simulink model "frft_qpsk_transceiver"  (R2025a)
settings: Solver=FixedStepDiscrete  StartTime=0.0  StopTime=1  RelTol=1e-3
PreLoadFcn:
  | % Add paths
  | addpath("dvb-s2/")
  | addpath("frft_filtering/")
  | addpath("gse")
  | 
  | 
  | 
  | 
  | setTxBurstLength = 10000;
  | txtmsg = ['Zynq radio HW/SW Co-design ÞÞÞÞ']; % Use only printable characters
  | 
  | %------------------------------------------------------------------------------------------------------
  | if ~isequal(size(txtmsg),[1 31])
  |     error('txtmsg must contain 31 characters');
  | end
  | 
  | [dataBits,msg] = zynqRadioHWSWQPSKgenHelloworldMsg(20); % generate 20 msgs for LUT
  | msgLUT = uint8(msg);
  | dataBitsLUT = dataBits(:);
  | Rsym                = 25e3;%1.92e6;
  | Config = zynqRadioHWSWQPSKTxRxParameters;
  | fs = Rsym*Config.SamplesPerSymbol;
  | word = [txtmsg newline];  % append a new line character to txtmsg
  | 
  | % The highest clock rate is 16 times the message character rate.
  | % As the message characters are fed at highest clock to FPGA
  | % repeat each character 16 times to maintain the message rate.
  | word = repelem(word.',16,1);
  | repeatTimes = ceil(setTxBurstLength/length(word));
  | inpData = complex(repmat(uint8(word),repeatTimes,1));
  | inUseTxBurstLength = length(inpData);
PostLoadFcn:
  | hScopeConfig = get_param([gcs '/HDL_QPSK/QPSK Tx Channel QPSK Rx/QPSK Rx/Frequency and Time Synchronizer/Symbol Synchronizer/No HDL/QPSK Receiver Eye Diagram'],'ScopeConfiguration');
  | hScopeConfig.OpenAtSimulationStart = false;
  | hScopeConfig.Visible = false;
  | clear hScopeConfig
InitFcn:
  | setTxBurstLength = 10000;
  | txtmsg = ['Zynq radio HW/SW Co-design ÞÞÞÞ']; % Use only printable characters
  | 
  | %------------------------------------------------------------------------------------------------------
  | if ~isequal(size(txtmsg),[1 31])
  |     error('txtmsg must contain 31 characters');
  | end
  | 
  | [dataBits,msg] = zynqRadioHWSWQPSKgenHelloworldMsg(20); % generate 20 msgs for LUT
  | msgLUT = uint8(msg);
  | dataBitsLUT = dataBits(:);
  | Rsym                = 25e3;%1.92e6;
  | Config = zynqRadioHWSWQPSKTxRxParameters;
  | fs = Rsym*Config.SamplesPerSymbol;
  | word = [txtmsg newline];  % append a new line character to txtmsg
  | 
  | % The highest clock rate is 16 times the message character rate.
  | % As the message characters are fed at highest clock to FPGA
  | % repeat each character 16 times to maintain the message rate.
  | word = repelem(word.',16,1);
  | repeatTimes = ceil(setTxBurstLength/length(word));
  | inpData = complex(repmat(uint8(word),repeatTimes,1));
  | inUseTxBurstLength = length(inpData);
undefined symbols (not defined in the file or in its folder): Add, dspblkCoreblockFVToolHelper, gcbh, Shift, unicode2native
libraries: hdlsllib x120, simulink x39, commseqgen3 x8, dsphdlsigops2 x4, whdledac x4, dsphdlfiltering2 x3, whdlutilities x3, dsphdlxfrm2 x2, dsphdlmathfun2 x2, commdigbbndpm3 x2, commchan3 x1, whdlmod x1
(part 5 of 5)

== system frft_qpsk_transceiver/Model Parameters/HDL_QPSK/QPSK Tx Channel QPSK Rx/QPSK Rx/Frequency and Time Synchronizer/Symbol Synchronizer/Rate Handle/FIFO ==
  in : Inport
  push : Inport  Port=2
  pop : Inport  Port=3
  reset : Inport  Port=4
  Delay1 : Delay  DelayLength=1
  Pop Counter : hdlsllib/Sources/HDL Counter  CountType=Count limited  CountInit=0  CountStep=1  CountMax=fifoSize -1  CountFromType=Initial value  CountFrom=0  CountResetPort=on  CountLoadPort=off  CountEnbPort=on  CountDirPort=off  CountHitOutputPort=off  CountDataType=Unsigned  CountWordLen=nextpow2(fifoSize)  CountFracLen=0  CountSampTime=1
  Push Counter : hdlsllib/Sources/HDL Counter  CountType=Count limited  CountInit=0  CountStep=1  CountMax=fifoSize -1  CountFromType=Initial value  CountFrom=0  CountResetPort=on  CountLoadPort=off  CountEnbPort=on  CountDirPort=off  CountHitOutputPort=off  CountDataType=Unsigned  CountWordLen=nextpow2(fifoSize)  CountFracLen=0  CountSampTime=1
  Simple Dual Port RAM : hdlsllib/HDL RAMs/Simple Dual Port RAM  ram_size=nextpow2(fifoSize)
  Validate Input Push Pop : Subsystem
  out : Outport
  numEntries : Outport  Port=2
  validPop : Outport  Port=3
  wires:
  Delay1/1 -> Push Counter/1, Pop Counter/1
  in/1 -> Simple Dual Port RAM/1
  reset/1 -> Validate Input Push Pop/1(rst), Delay1/1
  Validate Input Push Pop/2(valid pop) -> Pop Counter/2, validPop/1
  Validate Input Push Pop/1(valid push) -> Push Counter/2, Simple Dual Port RAM/3
  pop/1 -> Validate Input Push Pop/3(pop)
  push/1 -> Validate Input Push Pop/2(push)
  Pop Counter/1 -> Simple Dual Port RAM/4
  Push Counter/1 -> Simple Dual Port RAM/2
  Simple Dual Port RAM/1 -> out/1
  Validate Input Push Pop/3(numEntries) -> numEntries/1

== system frft_qpsk_transceiver/Model Parameters/HDL_QPSK/QPSK Tx Channel QPSK Rx/QPSK Tx/Bit Packetizer/Data Bits FIFO/No HDL/No HDL ==
  push : Inport
  full : Inport  Port=2
  ncount : Inport  Port=3
  empty : Inport  Port=4
  pop : Inport  Port=5
  Assertion : Assertion
  Assertion1 : Assertion
  Display : Display
  Logical Operator : Logic  Operator=NAND  AllPortsSameDT=off  OutDataTypeStr=boolean
  Logical Operator1 : Logic  Operator=NAND  AllPortsSameDT=off  OutDataTypeStr=boolean
  wires:
  Logical Operator1/1 -> Assertion1/1
  ncount/1 -> Display/1
  Logical Operator/1 -> Assertion/1
  pop/1 -> Logical Operator1/2
  full/1 -> Logical Operator/2
  empty/1 -> Logical Operator1/1
  push/1 -> Logical Operator/1

== system frft_qpsk_transceiver/Model Parameters/HDL_QPSK/QPSK Tx Channel QPSK Rx/QPSK Rx/Frequency and Time Synchronizer/Coarse Frequency Compensator/Coarse Frequency Estimator/Integrator/Reset Generator ==
  validIn : Inport
  Compare To Constant : simulink/Logic and Bit Operations/Compare To Constant  relop===  const=integAvgLen  OutDataTypeStr=boolean
  Delay1 : Delay  DelayLength=1
  Delay5 : Delay  DelayLength=1
  HDL Counter : hdlsllib/Sources/HDL Counter  CountType=Count limited  CountInit=0  CountStep=1  CountMax=integAvgLen  CountFromType=Initial value  CountFrom=0  CountResetPort=off  CountLoadPort=off  CountEnbPort=on  CountDirPort=off  CountHitOutputPort=off  CountDataType=Unsigned  CountWordLen=nextpow2(integAvgLen + 1)  CountFracLen=0  CountSampTime=1
  Logical Operator : Logic  AllPortsSameDT=off  OutDataTypeStr=boolean
  reset : Outport
  wires:
  Delay1/1 -> Logical Operator/1
  Delay5/1 -> Compare To Constant/1
  Logical Operator/1 -> reset/1
  validIn/1 -> HDL Counter/1, Delay1/1
  Compare To Constant/1 -> Logical Operator/2
  HDL Counter/1 -> Delay5/1

== system frft_qpsk_transceiver/Model Parameters/HDL_QPSK/QPSK Tx Channel QPSK Rx/QPSK Rx/Frequency and Time Synchronizer/PL Data Descrambler/PL Data Descrambler/PL Scrambler Gold Sequence Generator/Subsystem ==
  note: The initial output of these outports are set to 0 as this is an enabled subsystem
  reset : Inport
  Enable : EnablePort
  X PN Generator M_n : commseqgen3/PN Sequence Generator  poly='z^18+z^7+1'  ini_sta=[zeros(1,17) 1]  outBitMaskSource=Dialog parameter  shift=n  outVarSiz=off  maxOutSizeMode=Dialog parameter  maxOutSize=[10 1]  Ts=-1  sampPerFrame=1  reset=on  bitPackedOutputs=off  outDataType=boolean  numPackedBits=8  bitPackDataSigned=off  bitPackedOutDType=double
  X PN Generator M_nplus131072 : commseqgen3/PN Sequence Generator  poly='z^18+z^7+1'  ini_sta=[zeros(1,17) 1]  outBitMaskSource=Dialog parameter  shift=n+131072  outVarSiz=off  maxOutSizeMode=Dialog parameter  maxOutSize=[10 1]  Ts=-1  sampPerFrame=1  reset=on  bitPackedOutputs=off  outDataType=boolean  numPackedBits=8  bitPackDataSigned=off  bitPackedOutDType=double
  Y PN Generator M_0 : commseqgen3/PN Sequence Generator  poly='z^18 + z^10 + z^7 + z^5 + 1'  ini_sta=ones(1,18)  outBitMaskSource=Dialog parameter  shift=0  outVarSiz=off  maxOutSizeMode=Dialog parameter  maxOutSize=[10 1]  Ts=-1  sampPerFrame=1  reset=on  bitPackedOutputs=off  outDataType=boolean  numPackedBits=8  bitPackDataSigned=off  bitPackedOutDType=double
  Y PN Generator M_131072 : commseqgen3/PN Sequence Generator  poly='z^18 + z^10 + z^7 + z^5 + 1'  ini_sta=ones(1,18)  outBitMaskSource=Dialog parameter  shift=131072  outVarSiz=off  maxOutSizeMode=Dialog parameter  maxOutSize=[10 1]  Ts=-1  sampPerFrame=1  reset=on  bitPackedOutputs=off  outDataType=boolean  numPackedBits=8  bitPackDataSigned=off  bitPackedOutDType=double
  xMnp131072 : Outport  InitialOutput=0
  yM131072 : Outport  Port=2  InitialOutput=0
  xMn : Outport  Port=3  InitialOutput=0
  yM0 : Outport  Port=4  InitialOutput=0
  wires:
  X PN Generator M_nplus131072/1 -> xMnp131072/1
  Y PN Generator M_0/1 -> yM0/1
  reset/1 -> X PN Generator M_nplus131072/1, Y PN Generator M_0/1, X PN Generator M_n/1, Y PN Generator M_131072/1
  X PN Generator M_n/1 -> xMn/1
  Y PN Generator M_131072/1 -> yM131072/1

== system frft_qpsk_transceiver/Model Parameters/HDL_QPSK/QPSK Tx Channel QPSK Rx/QPSK Rx/Frequency and Time Synchronizer/Phase Ambiguity Estimation and Correction/Phase Ambiguity Corrector/Reciprocal/Function Impl ==
  switch : Inport
  LUTAddr : Inport  Port=2
  Delay{6..8,10,15..16} (6 alike) : Delay
  Delay9 : Delay  DelayLength=1
  LUT1 : LookupNDDirect  NumberOfTableDimensions=1  Table=LUT(:,1)  DiagnosticForOutOfRangeInput=Error
  LUT2 : LookupNDDirect  NumberOfTableDimensions=1  Table=LUT(:,2)  DiagnosticForOutOfRangeInput=Error
  Multiport Switch : MultiPortSwitch  DataPortOrder=Zero-based contiguous  Inputs=2  zeroidx=on  SaturateOnIntegerOverflow=off  InputSameDT=off
  functionValues : Outport
  wires:
  Multiport Switch/1 -> Delay9/1
  Delay6/1 -> LUT1/1
  Delay7/1 -> LUT2/1
  Delay8/1 -> Delay10/1
  switch/1 -> Delay8/1
  LUT1/1 -> Delay16/1
  LUT2/1 -> Delay15/1
  Delay9/1 -> functionValues/1
  Delay10/1 -> Multiport Switch/1
  Delay16/1 -> Multiport Switch/3
  Delay15/1 -> Multiport Switch/2
  LUTAddr/1 -> Delay6/1, Delay7/1

== system frft_qpsk_transceiver/Model Parameters/HDL_QPSK/QPSK Tx Channel QPSK Rx/QPSK Rx/Frequency and Time Synchronizer/Preamble Detector/Timing Adjust/No HDL/No HDL ==
  timingOffset : Inport
  Enable : EnablePort
  Data Type Conversion : DataTypeConversion  OutDataTypeStr=double  SaturateOnIntegerOverflow=off  RndMeth=Floor
  To Workspace : ToWorkspace  VariableName=simTimingOffset  SampleTime=-1
      settings: Save2DSignal=2-D array (concatenate along first dimension)
  wires:
  Data Type Conversion/1 -> To Workspace/1
  timingOffset/1 -> Data Type Conversion/1

== system frft_qpsk_transceiver/Model Parameters/HDL_QPSK/QPSK Tx Channel QPSK Rx/QPSK Rx/Frequency and Time Synchronizer/Preamble Detector/Timing Adjust/No HDL/No HDL1 ==
  frameNumber : Inport
  Enable : EnablePort
  Data Type Conversion : DataTypeConversion  OutDataTypeStr=double  SaturateOnIntegerOverflow=off  RndMeth=Floor
  To Workspace : ToWorkspace  VariableName=simSyncedPackets  SampleTime=-1
      settings: Save2DSignal=2-D array (concatenate along first dimension)
  wires:
  frameNumber/1 -> Data Type Conversion/1
  Data Type Conversion/1 -> To Workspace/1

== system frft_qpsk_transceiver/Model Parameters/HDL_QPSK/QPSK Tx Channel QPSK Rx/QPSK Rx/Frequency and Time Synchronizer/Symbol Synchronizer/Rate Handle/FIFO/Validate Input Push Pop ==
  rst : Inport
  push : Inport  Port=2
  pop : Inport  Port=3
  Compare To Constant : hdlsllib/Logic and Bit Operations/Compare To Constant  relop===  const=0  OutDataTypeStr=boolean
  Compare To Constant1 : hdlsllib/Logic and Bit Operations/Compare To Constant  relop===  const=fifoSize  OutDataTypeStr=boolean
  Constant : Constant  Value=true  SampleTime=-1
  Constant1 : Constant  Value=false  SampleTime=-1
  Delay : Delay  DelayLength=1
  Logical Operator1 : Logic  Operator=XOR  AllPortsSameDT=off  OutDataTypeStr=boolean
  Logical Operator2 : Logic  Operator=NOT  AllPortsSameDT=off  OutDataTypeStr=boolean
  Logical Operator{3..5,7,9} (5 alike) : Logic  AllPortsSameDT=off  OutDataTypeStr=boolean
  Logical Operator6 : Logic  Operator=NOT  AllPortsSameDT=off  OutDataTypeStr=boolean
  Logical Operator8 : Logic  Operator=NOT  AllPortsSameDT=off  OutDataTypeStr=boolean
  MATLAB Function : MATLAB Function  TreatAsAtomicUnit=on  mask{initVal=0, countToVal=fifoSize}
      mask prompts: initVal "Initial value:"; countToVal "Count to value:"
  No HDL : Subsystem
  Switch : Switch  Criteria=u2 ~= 0  SaturateOnIntegerOverflow=off  InputSameDT=off
  valid push : Outport
  valid pop : Outport  Port=2
  numEntries : Outport  Port=3
  wires:
  Logical Operator9/1 -> Logical Operator1/1, valid push/1
  Logical Operator2/1 -> Logical Operator9/2
  Logical Operator5/1 -> Logical Operator4/1
  Logical Operator8/1 -> Logical Operator5/2
  push/1 -> Logical Operator5/1, Logical Operator9/1
  Logical Operator1/1 -> MATLAB Function/2(enb)
  Logical Operator6/1 -> Logical Operator7/2
  Logical Operator7/1 -> Switch/2, valid pop/1, Logical Operator8/1, Logical Operator1/2
  Compare To Constant1/1 -> Logical Operator4/2
  Constant/1 -> Switch/3
  Logical Operator4/1 -> No HDL/1(pushFullFIFO), Logical Operator2/1  "push on full FIFO"
  Logical Operator3/1 -> No HDL/2(popEmptyFIFO), Logical Operator6/1  "pop on empty FIFO"
  Constant1/1 -> Switch/1
  MATLAB Function/1(count) -> Delay/1
  Switch/1 -> MATLAB Function/3(dir)
  pop/1 -> Logical Operator3/2, Logical Operator7/1
  Compare To Constant/1 -> Logical Operator3/1
  rst/1 -> MATLAB Function/1(rst)
  Delay/1 -> Compare To Constant1/1, numEntries/1, Compare To Constant/1

== system frft_qpsk_transceiver/Model Parameters/HDL_QPSK/QPSK Tx Channel QPSK Rx/QPSK Rx/Frequency and Time Synchronizer/Symbol Synchronizer/Rate Handle/FIFO/Validate Input Push Pop/No HDL ==
  pushFullFIFO : Inport
  popEmptyFIFO : Inport  Port=2
  Constant2 : Constant  Value=pushFullDiag  SampleTime=-1
  Constant3 : Constant  Value=popEmptyDiag  SampleTime=-1
  MATLAB Function : MATLAB Function  TreatAsAtomicUnit=on
  wires:
  Constant2/1 -> MATLAB Function/1(pushFullDiag)
  Constant3/1 -> MATLAB Function/2(popEmptyDiag)
  popEmptyFIFO/1 -> MATLAB Function/4(popEmpty)
  pushFullFIFO/1 -> MATLAB Function/3(pushFull)

== matlab function frft_qpsk_transceiver/Model Parameters/Channel & FRFT/Subsystem/frft_filter ==
  data: sigIn input; sigOut output; validIn input size=1; validOut output size=1; thresh parameter
% Function mock_frft_filter
% Use matlab FRFT implemention to filter on a frame wise basis

function [sigOut, validOut] = frft_filter( ...
                                    sigIn, validIn, ... % Ports
                                    thresh ...          % Params
                                    )
%#codegen

% Peak suppressoion
if (~validIn)
    sigOut = complex(zeros(size(sigIn)));
    validOut = false;
else 
    sig_reg = sigIn;

    stdthresh = std(sig_reg);


    % Look for area with high variance ->

    for xit = 1:length(sigIn)
        if abs(sig_reg(xit)) > thresh
            sig_reg(xit) = 0 + 0i;
        end
    end
    sigOut = sig_reg;
    validOut = true;
end



end

== matlab function frft_qpsk_transceiver/Model Parameters/Channel & FRFT/add_chirp ==
  data: sigIn input; sigOut output; validIn input boolean; chirpEn input boolean; validOut output boolean; fs parameter; T parameter; f0 parameter; f1 parameter; sir parameter
% Function add_chirp
% Combine input with chirp signal specified by mask params
% Signal is complex 12 bit integer stored within 16 bit int.
function [sigOut, validOut] = add_chirp( ...
                                sigIn, validIn, chirpEn, ... % Ports
                                fs, T, f0, f1, sir)...            % Parameters
%#codegen

% Setup registers
persistent t_reg sig_reg
if isempty(t_reg)
    % zero 
    t_reg = double(0); 
    sig_reg = complex(double(0));

end

% Pass through signal unless chirp enabled
if(~chirpEn)
    sigOut = complex(double(sigIn));
    validOut = validIn;
% Add Chirp Signal
else
    % Unless valid, just hold output value
    if (~validIn)
        sigOut = complex(double(sig_reg));
        validOut = false;
    % If valid, add chirp
    else 
        % Complex chirp
        sigOut = complex(double(add_chirp(complex(double(sigIn)),t_reg,fs, T, f0, f1, sir)));
        validOut = true;
        
        % Time update
        if (t_reg == T)
            t_reg = 0;
        else 
            t_reg = t_reg+1/fs;
        end
    end
    
end



end
% End add_chirp

== matlab function frft_qpsk_transceiver/Model Parameters/Channel & FRFT/Subsystem/frft_transform ==
  data: sigIn input; sigOut output; validIn input size=1; validOut output size=1; p input
function [sigOut, validOut] = frft_transform( ...
                                            sigIn, validIn, p ... % ports
                                            )
%#codegen
%FRFT_TRANSFORM Peak search in FRFT domain
%   1D Maximum peak search to identify optimum FRFT power
sigOut = sigIn;
validOut = validIn;

% If no valid input, only output 0.
if (~validIn)
    validOut = false;
    sigOut = zeros(size(sigIn));
    p_max = 0;

% ValidIn
else
    sig_reg = sigIn;
    sigOut = frft(sig_reg, p);
    sigOut(isnan(sigOut)) = 0;
    sigOut(isinf(sigOut)) = 0;

    validOut = true;
end




end
% END frft_transform

== matlab function frft_qpsk_transceiver/Model Parameters/Channel & FRFT/Subsystem/windowing ==
  data: sigIn input size=4000; sigOut output size=4000; validIn input size=1; validOut output size=1
function [sigOut, validOut] = window_sig( ...
                                            sigIn, validIn) ... % Ports % Params
%#codegen
%FRFT_TRANSFORM Peak search in FRFT domain
%   1D Maximum peak search to identify optimum FRFT power

% If no valid input, only output 0.
if (~validIn)
    validOut = false;
    sigOut = complex(squeeze(zeros(4000,1)));
% ValidIn
else

   
    window = complex(hamming(4000));
    sigOut = window.*sigIn;
    validOut = true;

end




end
% END frft_transform

== matlab function frft_qpsk_transceiver/Model Parameters/printData/MATLAB Function ==
  data: frm_start input; frm_end input; u input; msg_length parameter; frame_length parameter; frameOut output uint8 size=[1,frame_length]; frameValid output; msg_orig parameter
function [frameOut, frameValid] = printData(frm_start,frm_end,u, msg_length, frame_length, msg_orig)
%#codegen

% Byte Counter
persistent n

% Header (5 Bytes)
persistent header
persistent hmac
persistent frmmsg;

persistent frmReg


% HMAC (32 Bytes)

if isempty(n)
    header  = zeros(1,9,"uint8");
    hmac    = zeros(1,32,"uint8");
    n       = uint16(0);
    frmReg = zeros(1,frame_length,"uint8");

    frmmsg = zeros(1,msg_length);
end

frameOut = zeros(1,frame_length,"uint8");
frameValid = false;

 if frm_start
     fprintf("\nSTART =========\n");
     n=uint16(0);
     frmReg = zeros(1,frame_length,"uint8");
     frmmsg = zeros(1,length(msg_orig));
 end

if n<frame_length
    frmReg(n+1) = u;
end

if n < 8
    header(n+1) = u;
elseif n == 8
    fprintf("HEADER> ");
    fprintf("0x");
    for it = 1:2:8
        fprintf("%02X%02X ", header(it), header(it+1));
    end
    fprintf(" %02X \n", header(9));

    fprintf("MESSAGE> ");
% MESSAGE
elseif n < msg_length+8
    frmmsg(n-8) = u;
    u = bitand(u,0b01111111);
    if (u ~= 10) && ((u < 32) || (u > 192))
        u(:) = 94;  % print ^ for non printable characters except for newline 
    end
    fprintf('%c',char(u));
elseif n < msg_length+8+32
    fprintf("\n");
    hmac(n - msg_length - 8 + 1) = u;
end

if frm_end
 fprintf("HMAC> 0x");
 for it = 1:2:32
    fprintf("%02X%02X ", hmac(it), hmac(it+1));
 end
 
 ber = int2bit(frmmsg',8) ~= int2bit(msg_orig',8);
 ber = sum(ber);
 ber = ber / (msg_length*8);

 fprintf("\nMSG BER: %.3f",ber);

 fprintf("\nEND   =========\n");
 frameOut = frmReg;
 frameValid = true;
end




n = n + 1;

end

== matlab function frft_qpsk_transceiver/Model Parameters/HDL_QPSK/QPSK Tx Channel QPSK Rx/QPSK Tx/Bit Packetizer/Data Bits FIFO/No HDL/MATLAB Function ==
  data: wr input; full output; rd input; ncount output; empty output; dataBitsPerPacket parameter
function [full,ncount,empty] = fcn(wr,rd,dataBitsPerPacket)
%#codegen
     
    depth = dataBitsPerPacket*2 - 1;
    persistent count;
    if isempty(count)
        count = fi(0,0,nextpow2(depth),0,hdlfimath);
    end

    empty = (count == 0);
    full = (count > depth);
    ncount = count;

    if wr
        count(:) = count + 1;
    end
    if rd
        count(:) = count - 1;
    end

end

== matlab function frft_qpsk_transceiver/Model Parameters/HDL_QPSK/QPSK Tx Channel QPSK Rx/channel/add_chirp ==
  data: sigIn input; sigOut output; validIn input boolean; chirpEn input boolean; validOut output boolean; fs parameter; T parameter; f0 parameter; f1 parameter; sir parameter
% Function add_chirp
% Combine input with chirp signal specified by mask params
% Signal is complex 12 bit integer stored within 16 bit int.
function [sigOut, validOut] = add_chirp( ...
                                sigIn, validIn, chirpEn, ... % Ports
                                fs, T, f0, f1, sir)...            % Parameters
%#codegen

% Setup registers
persistent t_reg sig_reg
if isempty(t_reg)
    % zero 
    t_reg = double(0); 
    sig_reg = complex(double(0));

end

% Pass through signal unless chirp enabled
if(~chirpEn)
    sigOut = complex(double(sigIn));
    validOut = validIn;
% Add Chirp Signal
else
    % Unless valid, just hold output value
    if (~validIn)
        sigOut = complex(double(sig_reg));
        validOut = false;
    % If valid, add chirp
    else 
        % Complex chirp
        sigOut = complex(double(add_chirp(complex(double(sigIn)),t_reg,fs, T, f0, f1, sir)));
        validOut = true;
        
        % Time update
        if (t_reg == T)
            t_reg = 0;
        else 
            t_reg = t_reg+1/fs;
        end
    end
    
end



end
% End add_chirp

== matlab function frft_qpsk_transceiver/Model Parameters/HDL_QPSK/QPSK Tx Channel QPSK Rx/QPSK Tx/Bit Packetizer/Data Bits FIFO/RAM Frame Status Indicator ==
  data: push input; out output; pop input; dataBitsPerPacket parameter
function out = fcn(push,pop,dataBitsPerPacket)

   persistent pushCount popCount frameCount;
   if isempty(pushCount)
       pushCount = fi(0,0,nextpow2(dataBitsPerPacket),0,hdlfimath);
       frameCount = fi(0,0,2,0,hdlfimath);
       popCount = fi(0,0,nextpow2(dataBitsPerPacket),0,hdlfimath);
   end
   
   if (pushCount == dataBitsPerPacket-1) && push
       frameCount(:) = frameCount + 1;
   end
   if (popCount == dataBitsPerPacket-1) && pop
       frameCount(:) = frameCount - 1;
   end

   if push
       if pushCount == dataBitsPerPacket - 1
           pushCount(:) = 0;
       else
           pushCount(:) = pushCount + 1;
       end
   end

   if pop 
       if popCount == dataBitsPerPacket - 1
           popCount(:) = 0;
       else
           popCount(:) = popCount + 1;
       end
   end

   out = frameCount;

end

== matlab function frft_qpsk_transceiver/Model Parameters/HDL_QPSK/QPSK Tx Channel QPSK Rx/QPSK Rx/Frequency and Time Synchronizer/Packet Controller/MATLAB Function ==
  data: valid input; syncPulse input; out output
function out = fcn(valid,syncPulse)
%#codegen

  persistent Reg;
  if isempty(Reg)
      Reg = false;
  end
  
  out = Reg;
  
  if Reg && valid
      Reg = false;
  end
  
  if syncPulse
      Reg = true;
  end
  
end

== matlab function frft_qpsk_transceiver/Model Parameters/HDL_QPSK/QPSK Tx Channel QPSK Rx/QPSK Rx/Frequency and Time Synchronizer/Symbol Synchronizer/Rate Handle/FIFO/Validate Input Push Pop/MATLAB Function ==
  data: rst input; count output; enb input; dir input; initVal parameter; countToVal parameter
function count = hdlCounter(rst,enb,dir,initVal,countToVal)
%#codegen

persistent countReg

if(isempty(countReg))
    countReg = fi(initVal,0,nextpow2(countToVal+1),0);
end

if(rst)
    countReg(:) = initVal;
elseif(enb)
    if(dir)
        if(countReg==countToVal)
            countReg(:) = initVal;
        else
            countReg(:) = countReg+1;
        end
    else
        if(countReg==initVal)
            countReg(:) = countToVal;
        else
            countReg(:) = countReg-1;
        end
    end
end

count = countReg;

end

== matlab function frft_qpsk_transceiver/Model Parameters/HDL_QPSK/QPSK Tx Channel QPSK Rx/QPSK Tx/Bit Packetizer/Data Bits FIFO/MATLAB Function1 ==
  data: wr input; full output; rd input; dataBitsPerPacket parameter
function full = fcn(wr,rd,dataBitsPerPacket)
%#codegen
     
    depth = dataBitsPerPacket*2 - 1;
    persistent count;
    if isempty(count)
        count = fi(0,0,nextpow2(depth),0,hdlfimath);
    end

    if wr
        count(:) = count + 1;
    end
    if rd
        count(:) = count - 1;
    end

    full = (count > depth);

end

== matlab function frft_qpsk_transceiver/Model Parameters/HDL_QPSK/QPSK Tx Channel QPSK Rx/QPSK Rx/Frequency and Time Synchronizer/Packet Controller/sample discard controller ==
  data: dataIn input; validIn input; dataOut output; startIn input; endIn input; startOut output; endOut output; validOut output
function [dataOut,startOut,endOut,validOut] = controller(dataIn,validIn,startIn,endIn)
%#codegen

   persistent active dataOutReg validOutReg startOutReg endOutReg;
   if isempty(active)
      active  = false;
      dataOutReg = cast(0,'like',dataIn);
      validOutReg = false;
      startOutReg = false;
      endOutReg = false;
   end
   
   dataOut = dataOutReg;
   validOut = validOutReg;
   startOut = startOutReg;
   endOut = endOutReg;
   
   startOutReg = startIn;
   endOutReg = endIn;
   
   if startIn
       active = true;
   end
   
   if active
       dataOutReg(:) = dataIn;
       validOutReg = validIn;
   else
       dataOutReg(:) = 0;
       validOutReg = false;
   end
   
   if endIn
       if active 
           endOutReg = true;
       else
           endOutReg = false;
       end
       active = false;
   end
end

== matlab function frft_qpsk_transceiver/Model Parameters/HDL_QPSK/QPSK Tx Channel QPSK Rx/QPSK Rx/Frequency and Time Synchronizer/Symbol Synchronizer/Interpolation Control ==
  data: mu output; Delta input; Underflow output
function [mu,Underflow] = Interpolation_ctrl(Delta)
% Implementation of modulo-1 counter for interpolation control listed in
% Figure 8.4.19 of "Digital Communications - A Discrete-Time Approach"
% by Michael Rice. See design details in Chapter 8.4.3 of the same book.
% 
% Input:
%   Delta - Loop filter output. If loop is in lock, delta would be small
% Output:
%   Underflow - Indicator of counter underflow. This is the strobe signal
%               for downstream processing
%   mu - Difference between actual sampling instant and the optimal instant,
%        between zero and one
%#codegen

% countReg - Counter value delayed by 1 sample
% muReg - The estimated timing error normalized by half QPSK symbols

   mask = fi(1-2^(-10),1,11,10);
   
   persistent countReg underflowReg muReg;
   if isempty(countReg)
       countReg  = fi(0,1,11,10);
       muReg = fi(0,1,11,10);
       underflowReg = false;
   end
   
   
   Underflow = underflowReg;
   mu = muReg;   
   
   
   counter = bitand(mask,countReg)-Delta-fi(0.25,1,11,10); % decrementing counter
   
   % if countReg is a nonnegative number,
   % then mod(countReg,1) equals the fractional part of countReg
   if counter < 0
       underflowReg = true;
       muReg = bitshift(bitand(mask,countReg),2);
       countReg = fi(counter+1,1,11,10);% create underflow to counter
   else
       underflowReg = false;
       countReg = fi(counter,1,11,10);
   end
   


end

== matlab function frft_qpsk_transceiver/Model Parameters/HDL_QPSK/QPSK Tx Channel QPSK Rx/QPSK Rx/Frequency and Time Synchronizer/Preamble Detector/Correlator/ThresholdLimiter ==
  settings: fimath=hdlfimath
  data: x input; y output
function y = applyLowerLimit(x)
    % Apply a lower limit to the threshold.
    %#codegen
    
    % Threshold is computed by summing across 63 samples.
    % Set lower limit to be equivalent of all 63 samples
    % having their LSB set to 1 and all others set to 0. 
    lowerLimit = cast(0.01, 'like', x);
    
    if x < lowerLimit
        y = lowerLimit;
    else
        y = x;
    end
end

== matlab function frft_qpsk_transceiver/Model Parameters/Channel & FRFT/Subsystem/frft_peaksearch ==
  data: sigIn input size=4000; sigOut output size=4000; validIn input size=1; validOut output size=1; p_max output; n_iterations parameter; p_low parameter; p_high parameter
function [sigOut, validOut, p_max] = frft_peaksearch( ...
                                            sigIn, validIn, ... % Ports
                                            n_iterations, p_low, p_high)... % Params
%#codegen
%FRFT_TRANSFORM Peak search in FRFT domain
%   1D Maximum peak search to identify optimum FRFT power

% If no valid input, only output 0.
if (~validIn)
    validOut = false;
    sigOut = double(zeros(size(sigIn)));
    p_max = double(0);

% ValidIn
else
    sig_reg = complex(double(sigIn));

    % Do Peak Search:
    [p_opt, ~] = find_frft_peak(sig_reg,n_iterations, [p_low,p_high], false);
    p_max = double(p_opt);

    sigOut = frft(sig_reg, p_max);
    validOut = true;

end




end
% END frft_transform

== matlab function frft_qpsk_transceiver/Model Parameters/HDL_QPSK/QPSK Tx Channel QPSK Rx/QPSK Rx/Frequency and Time Synchronizer/Symbol Synchronizer/Rate Handle/FIFO/Validate Input Push Pop/No HDL/MATLAB Function ==
  data: pushFullDiag input; popEmptyDiag input; pushFull input; popEmpty input
function pushPopDiagnostics(pushFullDiag, popEmptyDiag, pushFull, popEmpty)
%#codegen


if(pushFull)
    switch pushFullDiag
        case 2
            warning('Push signal applied on full FIFO');
        case 3
            error('Push signal applied on full FIFO');
        otherwise
    end
end

if(popEmpty)
    switch popEmptyDiag
        case 2
            warning('Pop signal applied on empty FIFO');
        case 3
            error('Pop signal applied on empty FIFO');
        otherwise
    end
end

end
